simulink model "dx_hand_model"  (R2017b)
settings: Solver=ode3  StartTime=0.0  StopTime=inf  FixedStep=0.01  RelTol=1e-3  EnableMultiTasking=on
InitFcn:
  | cutFreq = 0.1; % T
  | sampleTime = 0.01;
  | filt = tf(1,[cutFreq 1]);
  | filt = c2d(filt,sampleTime);
  | 
  | cutFreq2 = 1;
  | filt2 = tf(1,[cutFreq2 1]);
  | filt2 = c2d(filt2,sampleTime);
  | 
  | cutFreq3 = 0.3;
  | filt3 = tf(1,[cutFreq3 1]);
  | filt3 = c2d(filt3,sampleTime);
  | 
  | update_param = 2;
  | 
  | ampliFactor = 1.60;
  | ampliFactorMiddle = 2.00;
  | ampliFactorDistal = 1;
  | 
  | % Set Hand Address
  | % RightHandAddress = '10.100.39.144';
  | RightHandAddress = '10.24.4.91';
  | Verosim = '10.100.39.22'
  | LeftHandAddress = '10.100.39.22'
  | 
  | max_force = 24; % Newton
model workspace (MAT data in the model file):
  SL_ROS_VariableLengthArrays_MaxSizes : struct (value not decoded)
libraries: robotlib x136, simulink_extras x27, simulink x16, etargetslib x2, dspnetwork x2
(part 2 of 19)

== system dx_hand_model/Pinky Finger/Choose_ ==
  pos : Inport
  force : Inport  Port=2
  Data Type Conversion1 : DataTypeConversion  OutDataTypeStr=single
  Get Parameter3 : robotlib/Get Parameter  SourceLibraryInfo=This block requires Robotics System Toolbox  ParameterSource=Specify your own  ParameterName=/hand_exo/pinky/modes/type  ParameterType=double  ParameterMaxArrayLength=16  ParameterInitialValue=1.0  SampleTime=update_param  ShowErrorCodeOutput=off  ModelName=dx_hand_model  BlockId=ParamGet_dx_hand_model_4579
      settings: SourceProductName=Robotics System Toolbox  SourceProductBaseCode=RO
  Rate Transition : RateTransition
  Switch : Switch  Criteria=u2 > Threshold
  out : Outport
  wires:
  Switch/1 -> out/1
  Data Type Conversion1/1 -> Switch/2
  Rate Transition/1 -> Data Type Conversion1/1
  Get Parameter3/1 -> Rate Transition/1
  force/1 -> Switch/3
  pos/1 -> Switch/1

== system dx_hand_model/Pinky Finger/Jacobian Calculation ==
  note: this jacobian has all lenght expressed in meters
  note: this jacobian has all lenght expressed in mm
  Pose : Inport
  Sensor : Inport  Port=2
  Measurements : Inport  Port=3
  Data Type Conversion1 : DataTypeConversion  OutDataTypeStr=single
  Data Type Conversion2 : DataTypeConversion  OutDataTypeStr=single
  Display1 : Display
  Display7 : Display
  Manual Switch : ManualSwitch
  Pinky Jacobian : MATLAB Function  TreatAsAtomicUnit=on  SystemSampleTime=0.01
  "Pinky Jacobian " : MATLAB Function  TreatAsAtomicUnit=on  SystemSampleTime=0.01
  Unit Delay1 : UnitDelay  InitialCondition=-1  SampleTime=0.01
  Unit Delay3 : UnitDelay  InitialCondition=[0;2.3]  SampleTime=0.01
  Jacobian : Outport
  wires:
  Pinky Jacobian/1(JTcomp) -> Manual Switch/2, Display7/1
  Data Type Conversion1/1 -> Pinky Jacobian/5(J22_old)
  Pinky Jacobian/2(q_next) -> Unit Delay3/1
  Data Type Conversion2/1 -> Pinky Jacobian/4(q_pr)
  Pinky Jacobian/3(J22_ol) -> Unit Delay1/1
  Unit Delay3/1 -> Data Type Conversion2/1
  Unit Delay1/1 -> Data Type Conversion1/1
  Measurements/1 -> "Pinky Jacobian "/3(measurements), Pinky Jacobian/3(measurements)
  Sensor/1 -> "Pinky Jacobian "/2(sensor), Pinky Jacobian/2(sensor)
  "Pinky Jacobian "/1(JTcomp) -> Display1/1, Manual Switch/1
  Pose/1 -> "Pinky Jacobian "/1(pose), Pinky Jacobian/1(pose)
  Manual Switch/1 -> Jacobian/1

== system dx_hand_model/Pinky Finger/Pose Generator ==
  Angular Potentiometer : Subsystem
  Constant : Constant
  Constant3 : Constant  Value=0
  Display : Display
  Display1 : Display
  Display3 : Display
  Linear Potentiometer : Subsystem
  Manual Switch : ManualSwitch  CurrentSetting=0
  Mux1 : Mux  Inputs=2
  Parametri Ring : Subsystem
  Pinky Direct Kinematics : MATLAB Function  TreatAsAtomicUnit=on
  Pinky Parameters : Subsystem
  Rate Transition : RateTransition
  Record : Subsystem
  Saturation2 : Saturate  UpperLimit=1000  LowerLimit=0
  Saturation3 : Saturate  UpperLimit=1000  LowerLimit=0
  Pose : Outport
  Sensors : Outport  Port=2
  Measurements : Outport  Port=3
  tag scope: PinkyPot1=global
  wires:
  Pinky Direct Kinematics/1(y) -> Pose/1, Record/3(output)
  Manual Switch/1 -> Record/Enable
  Angular Potentiometer/1(Deg) -> Display3/1
  [PinkyRotPot] -> Angular Potentiometer/1(ADC)
  [PinkyFlexLinPot] -> Linear Potentiometer/1(ADC)
  Saturation2/1 -> [PinkyPot1], Mux1/1
  Constant/1 -> Manual Switch/1
  Constant3/1 -> Manual Switch/2
  Angular Potentiometer/2(Rad) -> Display1/1, Saturation3/1
  Linear Potentiometer/1(mm) -> Display/1, Saturation2/1
  Mux1/1 -> Sensors/1, Record/1(input), Pinky Direct Kinematics/1(u)
  Saturation3/1 -> Mux1/2
  Pinky Parameters/1(to Direct Kin) -> Pinky Direct Kinematics/2(measurements), Measurements/1, Record/2(param)
  Parametri Ring/1(Par_5) -> Rate Transition/1
  Rate Transition/1 -> Pinky Parameters/1(Par5)

== system dx_hand_model/Pinky Finger/Position-Force Architecture ==
  Jacobian : Inport
  Classic_Static_Problem : MATLAB Function  TreatAsAtomicUnit=on
  Display6 : Display
  Optimized_Static_Problem : MATLAB Function  TreatAsAtomicUnit=on
  Position Force Basic Architecture : Subsystem
  Subsystem : Subsystem
  Feedforward Force : Outport
  wires:
  Position Force Basic Architecture/1(force_vec) -> Classic_Static_Problem/2(force_vector), Optimized_Static_Problem/2(force_vector)
  Jacobian/1 -> Classic_Static_Problem/1(Jcomponents), Optimized_Static_Problem/1(Jcomponents)
  Subsystem/1(J_out) -> Feedforward Force/1, Display6/1
  Optimized_Static_Problem/1(y) -> Subsystem/1(optim)
  Classic_Static_Problem/1(y) -> Subsystem/2(classic)

== system dx_hand_model/Pinky Finger/Position-Position ==
  Jacobian : Inport
  Classic_Static_Problem : MATLAB Function  TreatAsAtomicUnit=on
  Discrete Derivative{,1..3} (4 alike) : simulink/Discrete/Discrete Derivative  gainval=1.0  ICPrevScaledInput=0.0  OutMin=[]  OutMax=[]  OutDataType=fixdt(1, 16)  OutScaling=2^-10  DoSatur=off
  Gain : Gain  Gain=1.3588
  Mux : Mux  Inputs=2
  Mux1 : Mux  Inputs=2
  Optimized_Static_Problem : MATLAB Function  TreatAsAtomicUnit=on
  Pre-Proc : Subsystem
  Saturation3 : Saturate  UpperLimit=0.80  LowerLimit=0
  Saturation4 : Saturate  UpperLimit=1.33  LowerLimit=0
  Sum{,1,3..4} (4 alike) : Sum  Inputs=|+-
  Sum2 : Sum  Inputs=|++
  active : Subsystem
  active1 : Subsystem
  setGain : Subsystem
  "setGain " : Subsystem
  setGain 1 : Subsystem
  setGain 2 : Subsystem
  rate : Outport
  wires:
  [act_Pinky] -> Gain/1, Discrete Derivative2/1, Sum/1
  Sum/1 -> setGain/1(in)
  "setGain "/1(out) -> Mux/2
  setGain/1(out) -> Mux/1
  [SchunkPinkyFingerDistal] -> Saturation4/1
  Mux/1 -> Sum2/1
  Mux1/1 -> Sum2/2
  Sum2/1 -> Optimized_Static_Problem/2(force_vector), Classic_Static_Problem/2(operational_space)
  [SchunkPinkyFingerProximal] -> Saturation3/1
  Saturation3/1 -> Sum/2, Discrete Derivative/1
  Saturation4/1 -> Sum1/2, Discrete Derivative1/1
  Gain/1 -> Discrete Derivative3/1, Sum1/1
  Jacobian/1 -> Optimized_Static_Problem/1(Jcomponents), Classic_Static_Problem/1(Jcomponents)
  Sum1/1 -> "setGain "/1(in)
  Sum3/1 -> setGain 1/1(in)
  Sum4/1 -> setGain 2/1(in)
  setGain 1/1(out) -> Mux1/1
  setGain 2/1(out) -> Mux1/2
  Optimized_Static_Problem/1(y) -> Pre-Proc/1(yes)
  Classic_Static_Problem/1(rate) -> Pre-Proc/2(no)
  Pre-Proc/1(out) -> rate/1
  Discrete Derivative/1 -> Sum3/2
  Discrete Derivative1/1 -> Sum4/2
  Discrete Derivative2/1 -> active/1(in)
  active/1(out) -> Sum3/1
  Discrete Derivative3/1 -> active1/1(in)
  active1/1(out) -> Sum4/1

== system dx_hand_model/Pinky Finger/Pre-Proc ==
  in : Inport
  Data Type Conversion1 : DataTypeConversion  OutDataTypeStr=single
  Data Type Conversion2 : DataTypeConversion  OutDataTypeStr=single
  Filt 4 : DiscreteTransferFcn  Numerator=filt2.Numerator{1,1}  Denominator=filt2.Denominator{1,1}  SampleTime=0.01
  Get Parameter3 : robotlib/Get Parameter  SourceLibraryInfo=This block requires Robotics System Toolbox  ParameterSource=Specify your own  ParameterName=/hand_exo/pinky/j_f  ParameterType=double  ParameterMaxArrayLength=16  ParameterInitialValue=1.0  SampleTime=update_param  ShowErrorCodeOutput=on  ModelName=dx_hand_model  BlockId=ParamGet_dx_hand_model_4804
      settings: SourceProductName=Robotics System Toolbox  SourceProductBaseCode=RO
  "IsNan " : MATLAB Function  TreatAsAtomicUnit=on
  Memory : Memory  InitialCondition=[0,0,0,0]
  Rate Transition : RateTransition
  Switch : Switch  Criteria=u2 > Threshold
  out : Outport
  wires:
  Get Parameter3/1 -> Rate Transition/1
  Rate Transition/1 -> Data Type Conversion1/1
  Data Type Conversion1/1 -> Switch/2
  Filt 4/1 -> Switch/1
  Switch/1 -> out/1
  Memory/1 -> Data Type Conversion2/1
  in/1 -> "IsNan "/1(Jin)
  Data Type Conversion2/1 -> "IsNan "/2(J_k1)
  "IsNan "/1(J) -> Switch/3, Filt 4/1, Memory/1

== system dx_hand_model/Pinky Finger/setGain ==
  in : Inport
  Data Type Conversion1 : DataTypeConversion  OutDataTypeStr=single
  Get Parameter3 : robotlib/Get Parameter  SourceLibraryInfo=This block requires Robotics System Toolbox  ParameterSource=Specify your own  ParameterName=/hand_exo/pinky/schunk_gains/prox  ParameterType=double  ParameterMaxArrayLength=16  ParameterInitialValue=1.0  SampleTime=update_param  ShowErrorCodeOutput=off  ModelName=dx_hand_model  BlockId=ParamGet_dx_hand_model_4815
      settings: SourceProductName=Robotics System Toolbox  SourceProductBaseCode=RO
  Product : Product
  Rate Transition : RateTransition
  out : Outport
  wires:
  Product/1 -> out/1
  Data Type Conversion1/1 -> Product/1
  in/1 -> Product/2
  Rate Transition/1 -> Data Type Conversion1/1
  Get Parameter3/1 -> Rate Transition/1

== system dx_hand_model/Pinky Finger/setGain1 ==
  in : Inport
  Data Type Conversion1 : DataTypeConversion  OutDataTypeStr=single
  Get Parameter3 : robotlib/Get Parameter  SourceLibraryInfo=This block requires Robotics System Toolbox  ParameterSource=Specify your own  ParameterName=/hand_exo/pinky/schunk_gains/dist  ParameterType=double  ParameterMaxArrayLength=16  ParameterInitialValue=1.0  SampleTime=update_param  ShowErrorCodeOutput=off  ModelName=dx_hand_model  BlockId=ParamGet_dx_hand_model_4822
      settings: SourceProductName=Robotics System Toolbox  SourceProductBaseCode=RO
  Product : Product
  Rate Transition : RateTransition
  out : Outport
  wires:
  Product/1 -> out/1
  Data Type Conversion1/1 -> Product/1
  in/1 -> Product/2
  Rate Transition/1 -> Data Type Conversion1/1
  Get Parameter3/1 -> Rate Transition/1

== system dx_hand_model/Pinky Finger/setGain2 ==
  in : Inport
  Data Type Conversion1 : DataTypeConversion  OutDataTypeStr=single
  Get Parameter3 : robotlib/Get Parameter  SourceLibraryInfo=This block requires Robotics System Toolbox  ParameterSource=Specify your own  ParameterName=/hand_exo/pinky/modes/saturator  ParameterType=double  ParameterMaxArrayLength=16  ParameterInitialValue=-1.0  SampleTime=update_param  ShowErrorCodeOutput=off  ModelName=dx_hand_model  BlockId=ParamGet_dx_hand_model_4829
      settings: SourceProductName=Robotics System Toolbox  SourceProductBaseCode=RO
  Rate Transition : RateTransition
  Saturation1 : Saturate  UpperLimit=max_force  LowerLimit=-max_force
  Saturation2 : Saturate  UpperLimit=0  LowerLimit=-max_force
  Switch : Switch  Criteria=u2 > Threshold
  out : Outport
  wires:
  Switch/1 -> out/1
  Data Type Conversion1/1 -> Switch/2
  Rate Transition/1 -> Data Type Conversion1/1
  Get Parameter3/1 -> Rate Transition/1
  in/1 -> Saturation1/1, Saturation2/1
  Saturation1/1 -> Switch/1
  Saturation2/1 -> Switch/3

== system dx_hand_model/Ring Finger /Active ==
  in : Inport
  Constant : Constant  Value=0  OutDataTypeStr=single
  Data Type Conversion1 : DataTypeConversion  OutDataTypeStr=single
  Get Parameter3 : robotlib/Get Parameter  SourceLibraryInfo=This block requires Robotics System Toolbox  ParameterSource=Specify your own  ParameterName=/hand_exo/ring/modes/ff_active  ParameterType=double  ParameterMaxArrayLength=16  ParameterInitialValue=1.0  SampleTime=update_param  ShowErrorCodeOutput=off  ModelName=dx_hand_model  BlockId=ParamGet_dx_hand_model_4879
      settings: SourceProductName=Robotics System Toolbox  SourceProductBaseCode=RO
  Rate Transition : RateTransition
  Switch : Switch  Criteria=u2 > Threshold
  out : Outport
  wires:
  Switch/1 -> out/1
  Data Type Conversion1/1 -> Switch/2
  Rate Transition/1 -> Data Type Conversion1/1
  Get Parameter3/1 -> Rate Transition/1
  in/1 -> Switch/1
  Constant/1 -> Switch/3

== system dx_hand_model/Ring Finger /Choose ==
  theoretical : Inport
  empiric : Inport  Port=2
  Data Type Conversion1 : DataTypeConversion  OutDataTypeStr=single
  Get Parameter3 : robotlib/Get Parameter  SourceLibraryInfo=This block requires Robotics System Toolbox  ParameterSource=Specify your own  ParameterName=/hand_exo/ring/modes/theor  ParameterType=double  ParameterMaxArrayLength=16  ParameterInitialValue=-1.0  SampleTime=update_param  ShowErrorCodeOutput=off  ModelName=dx_hand_model  BlockId=ParamGet_dx_hand_model_4903
      settings: SourceProductName=Robotics System Toolbox  SourceProductBaseCode=RO
  Rate Transition : RateTransition
  Switch : Switch  Criteria=u2 > Threshold
  out : Outport
  wires:
  Switch/1 -> out/1
  Data Type Conversion1/1 -> Switch/2
  Rate Transition/1 -> Data Type Conversion1/1
  Get Parameter3/1 -> Rate Transition/1
  empiric/1 -> Switch/3
  theoretical/1 -> Switch/1

== system dx_hand_model/Ring Finger /Choose_ ==
  pos : Inport
  force : Inport  Port=2
  Data Type Conversion1 : DataTypeConversion  OutDataTypeStr=single
  Get Parameter3 : robotlib/Get Parameter  SourceLibraryInfo=This block requires Robotics System Toolbox  ParameterSource=Specify your own  ParameterName=/hand_exo/ring/modes/type  ParameterType=double  ParameterMaxArrayLength=16  ParameterInitialValue=1.0  SampleTime=update_param  ShowErrorCodeOutput=off  ModelName=dx_hand_model  BlockId=ParamGet_dx_hand_model_4283
      settings: SourceProductName=Robotics System Toolbox  SourceProductBaseCode=RO
  Rate Transition : RateTransition
  Switch : Switch  Criteria=u2 > Threshold
  out : Outport
  wires:
  Switch/1 -> out/1
  Data Type Conversion1/1 -> Switch/2
  Rate Transition/1 -> Data Type Conversion1/1
  Get Parameter3/1 -> Rate Transition/1
  force/1 -> Switch/3
  pos/1 -> Switch/1

== system dx_hand_model/Ring Finger /Jacobian Calculation ==
  note: this jacobian has all lenght expressed in meters
  note: this jacobian has all lenght expressed in mm
  Pose : Inport
  Sensor : Inport  Port=2
  Measurements : Inport  Port=3
  Data Type Conversion1 : DataTypeConversion  OutDataTypeStr=single
  Data Type Conversion2 : DataTypeConversion  OutDataTypeStr=single
  Display1 : Display
  Display7 : Display
  Manual Switch : ManualSwitch
  Ring Jacobian : MATLAB Function  TreatAsAtomicUnit=on  SystemSampleTime=0.01
  "Ring Jacobian " : MATLAB Function  TreatAsAtomicUnit=on  SystemSampleTime=0.01
  Unit Delay1 : UnitDelay  InitialCondition=-1  SampleTime=0.01
  Unit Delay3 : UnitDelay  InitialCondition=[0;2.3]  SampleTime=0.01
  Jacobian : Outport
  wires:
  Ring Jacobian/1(JTcomp) -> Manual Switch/2, Display7/1
  Data Type Conversion1/1 -> Ring Jacobian/5(J22_old)
  Ring Jacobian/2(q_next) -> Unit Delay3/1
  Data Type Conversion2/1 -> Ring Jacobian/4(q_pr)
  Ring Jacobian/3(J22_ol) -> Unit Delay1/1
  Unit Delay3/1 -> Data Type Conversion2/1
  Unit Delay1/1 -> Data Type Conversion1/1
  Measurements/1 -> "Ring Jacobian "/3(measurements), Ring Jacobian/3(measurements)
  Sensor/1 -> "Ring Jacobian "/2(sensor), Ring Jacobian/2(sensor)
  "Ring Jacobian "/1(JTcomp) -> Display1/1, Manual Switch/1
  Pose/1 -> "Ring Jacobian "/1(pose), Ring Jacobian/1(pose)
  Manual Switch/1 -> Jacobian/1

== system dx_hand_model/Ring Finger /Pose Generator ==
  Angular Potentiometer : Subsystem
  Constant : Constant
  Constant3 : Constant  Value=0
  Display : Display
  Display1 : Display
  Display3 : Display
  Linear Potentiometer : Subsystem
  Manual Switch : ManualSwitch  CurrentSetting=0
  Mux1 : Mux  Inputs=2
  Parametri Ring : Subsystem
  Rate Transition : RateTransition
  Record : Subsystem
  Ring Direct Kinematics : MATLAB Function  TreatAsAtomicUnit=on
  Ring Parameters : Subsystem
  Saturation2 : Saturate  UpperLimit=1000  LowerLimit=0
  Saturation3 : Saturate  UpperLimit=1000  LowerLimit=0
  Pose : Outport
  Sensors : Outport  Port=2
  Measurements : Outport  Port=3
  tag scope: RingPot1=global
  wires:
  Ring Direct Kinematics/1(y) -> Pose/1, Record/3(output)
  Manual Switch/1 -> Record/Enable
  Angular Potentiometer/1(Deg) -> Display3/1
  [RingRotPot] -> Angular Potentiometer/1(ADC)
  [RingFlexLinPot] -> Linear Potentiometer/1(ADC)
  Saturation2/1 -> [RingPot1], Mux1/1
  Constant/1 -> Manual Switch/1
  Constant3/1 -> Manual Switch/2
  Angular Potentiometer/2(Rad) -> Display1/1, Saturation3/1
  Linear Potentiometer/1(mm) -> Display/1, Saturation2/1
  Mux1/1 -> Sensors/1, Record/1(input), Ring Direct Kinematics/1(u)
  Saturation3/1 -> Mux1/2
  Ring Parameters/1(to Direct Kin) -> Ring Direct Kinematics/2(measurements), Measurements/1, Record/2(param)
  Parametri Ring/1(Par_5) -> Rate Transition/1
  Rate Transition/1 -> Ring Parameters/1(Par5)

== system dx_hand_model/Ring Finger /Position-Force Architecture ==
  Jacobian : Inport
  Classic_Static_Problem : MATLAB Function  TreatAsAtomicUnit=on
  Display6 : Display
  Optimized_Static_Problem : MATLAB Function  TreatAsAtomicUnit=on
  Position Force Basic Architecture : Subsystem
  Subsystem : Subsystem
  Feedforward Force : Outport
  wires:
  Position Force Basic Architecture/1(force_vec) -> Classic_Static_Problem/2(force_vector), Optimized_Static_Problem/2(force_vector)
  Jacobian/1 -> Classic_Static_Problem/1(Jcomponents), Optimized_Static_Problem/1(Jcomponents)
  Subsystem/1(J_out) -> Feedforward Force/1, Display6/1
  Optimized_Static_Problem/1(y) -> Subsystem/1(optim)
  Classic_Static_Problem/1(y) -> Subsystem/2(classic)

== system dx_hand_model/Ring Finger /Position-Position ==
  Jacobian : Inport
  Classic_Static_Problem : MATLAB Function  TreatAsAtomicUnit=on
  Discrete Derivative{,1..3} (4 alike) : simulink/Discrete/Discrete Derivative  gainval=1.0  ICPrevScaledInput=0.0  OutMin=[]  OutMax=[]  OutDataType=fixdt(1, 16)  OutScaling=2^-10  DoSatur=off
  Gain : Gain  Gain=1.3588
  Mux : Mux  Inputs=2
  Mux1 : Mux  Inputs=2
  Optimized_Static_Problem : MATLAB Function  TreatAsAtomicUnit=on
  Pre-Proc : Subsystem
  Saturation3 : Saturate  UpperLimit=0.80  LowerLimit=0
  Saturation4 : Saturate  UpperLimit=1.33  LowerLimit=0
  Sum{,1,3..4} (4 alike) : Sum  Inputs=|+-
  Sum2 : Sum  Inputs=|++
  active : Subsystem
  active1 : Subsystem
  setGain : Subsystem
  "setGain " : Subsystem
  setGain 1 : Subsystem
  setGain 2 : Subsystem
  rate : Outport
  wires:
  [act_Ring] -> Gain/1, Discrete Derivative2/1, Sum/1
  Sum/1 -> setGain/1(in)
  "setGain "/1(out) -> Mux/2
  setGain/1(out) -> Mux/1
  [SchunkRingFingerDistal] -> Saturation4/1
  Mux/1 -> Sum2/1
  Mux1/1 -> Sum2/2
  Sum2/1 -> Optimized_Static_Problem/2(force_vector), Classic_Static_Problem/2(operational_space)
  [SchunkRingFingerProximal] -> Saturation3/1
  Saturation3/1 -> Sum/2, Discrete Derivative/1
  Saturation4/1 -> Sum1/2, Discrete Derivative1/1
  Gain/1 -> Discrete Derivative3/1, Sum1/1
  Jacobian/1 -> Optimized_Static_Problem/1(Jcomponents), Classic_Static_Problem/1(Jcomponents)
  Sum1/1 -> "setGain "/1(in)
  Sum3/1 -> setGain 1/1(in)
  Sum4/1 -> setGain 2/1(in)
  setGain 1/1(out) -> Mux1/1
  setGain 2/1(out) -> Mux1/2
  Optimized_Static_Problem/1(y) -> Pre-Proc/1(yes)
  Classic_Static_Problem/1(rate) -> Pre-Proc/2(no)
  Pre-Proc/1(out) -> rate/1
  Discrete Derivative/1 -> Sum3/2
  Discrete Derivative1/1 -> Sum4/2
  Discrete Derivative2/1 -> active/1(in)
  active/1(out) -> Sum3/1
  Discrete Derivative3/1 -> active1/1(in)
  active1/1(out) -> Sum4/1

== system dx_hand_model/Ring Finger /Pre-Proc ==
  in : Inport
  Data Type Conversion1 : DataTypeConversion  OutDataTypeStr=single
  Data Type Conversion2 : DataTypeConversion  OutDataTypeStr=single
  Filt 4 : DiscreteTransferFcn  Numerator=filt2.Numerator{1,1}  Denominator=filt2.Denominator{1,1}  SampleTime=0.01
  Get Parameter3 : robotlib/Get Parameter  SourceLibraryInfo=This block requires Robotics System Toolbox  ParameterSource=Specify your own  ParameterName=/hand_exo/ring/j_f  ParameterType=double  ParameterMaxArrayLength=16  ParameterInitialValue=1.0  SampleTime=update_param  ShowErrorCodeOutput=on  ModelName=dx_hand_model  BlockId=ParamGet_dx_hand_model_4518
      settings: SourceProductName=Robotics System Toolbox  SourceProductBaseCode=RO
  "IsNan " : MATLAB Function  TreatAsAtomicUnit=on
  Memory : Memory  InitialCondition=[0,0,0,0]
  Rate Transition : RateTransition
  Switch : Switch  Criteria=u2 > Threshold
  out : Outport
  wires:
  Get Parameter3/1 -> Rate Transition/1
  Rate Transition/1 -> Data Type Conversion1/1
  Data Type Conversion1/1 -> Switch/2
  Filt 4/1 -> Switch/1
  Switch/1 -> out/1
  Memory/1 -> Data Type Conversion2/1
  in/1 -> "IsNan "/1(Jin)
  Data Type Conversion2/1 -> "IsNan "/2(J_k1)
  "IsNan "/1(J) -> Switch/3, Filt 4/1, Memory/1

== system dx_hand_model/Ring Finger /setGain ==
  in : Inport
  Data Type Conversion1 : DataTypeConversion  OutDataTypeStr=single
  Get Parameter3 : robotlib/Get Parameter  SourceLibraryInfo=This block requires Robotics System Toolbox  ParameterSource=Specify your own  ParameterName=/hand_exo/ring/schunk_gains/prox  ParameterType=double  ParameterMaxArrayLength=16  ParameterInitialValue=1.0  SampleTime=update_param  ShowErrorCodeOutput=off  ModelName=dx_hand_model  BlockId=ParamGet_dx_hand_model_4529
      settings: SourceProductName=Robotics System Toolbox  SourceProductBaseCode=RO
  Product : Product
  Rate Transition : RateTransition
  out : Outport
  wires:
  Product/1 -> out/1
  Data Type Conversion1/1 -> Product/1
  in/1 -> Product/2
  Rate Transition/1 -> Data Type Conversion1/1
  Get Parameter3/1 -> Rate Transition/1

== system dx_hand_model/Ring Finger /setGain1 ==
  in : Inport
  Data Type Conversion1 : DataTypeConversion  OutDataTypeStr=single
  Get Parameter3 : robotlib/Get Parameter  SourceLibraryInfo=This block requires Robotics System Toolbox  ParameterSource=Specify your own  ParameterName=/hand_exo/ring/schunk_gains/dist  ParameterType=double  ParameterMaxArrayLength=16  ParameterInitialValue=1.0  SampleTime=update_param  ShowErrorCodeOutput=off  ModelName=dx_hand_model  BlockId=ParamGet_dx_hand_model_4536
      settings: SourceProductName=Robotics System Toolbox  SourceProductBaseCode=RO
  Product : Product
  Rate Transition : RateTransition
  out : Outport
  wires:
  Product/1 -> out/1
  Data Type Conversion1/1 -> Product/1
  in/1 -> Product/2
  Rate Transition/1 -> Data Type Conversion1/1
  Get Parameter3/1 -> Rate Transition/1

== system dx_hand_model/Ring Finger /setGain2 ==
  in : Inport
  Data Type Conversion1 : DataTypeConversion  OutDataTypeStr=single
  Get Parameter3 : robotlib/Get Parameter  SourceLibraryInfo=This block requires Robotics System Toolbox  ParameterSource=Specify your own  ParameterName=/hand_exo/ring/modes/saturator  ParameterType=double  ParameterMaxArrayLength=16  ParameterInitialValue=-1.0  SampleTime=update_param  ShowErrorCodeOutput=off  ModelName=dx_hand_model  BlockId=ParamGet_dx_hand_model_4543
      settings: SourceProductName=Robotics System Toolbox  SourceProductBaseCode=RO
  Rate Transition : RateTransition
  Saturation1 : Saturate  UpperLimit=max_force  LowerLimit=-max_force
  Saturation2 : Saturate  UpperLimit=0  LowerLimit=-max_force
  Switch : Switch  Criteria=u2 > Threshold
  out : Outport
  wires:
  Switch/1 -> out/1
  Data Type Conversion1/1 -> Switch/2
  Rate Transition/1 -> Data Type Conversion1/1
  Get Parameter3/1 -> Rate Transition/1
  in/1 -> Saturation1/1, Saturation2/1
  Saturation1/1 -> Switch/1
  Saturation2/1 -> Switch/3

== system dx_hand_model/Send to Schunk/Enable ==
  "Automatic " : ManualSwitch  CurrentSetting=0
  Blank Message1 : robotlib/Blank Message  SourceLibraryInfo=This block requires Robotics System Toolbox  messageType=std_msgs/Bool  SampleTime=inf
      settings: SourceProductBaseCode=RO
  Bus Assignment2 : BusAssignment  AssignedSignals=Data
  Bus Selector : BusSelector  OutputSignals=Data
  Constant : Constant  Value=0  OutDataTypeStr=boolean
  Constant1 : Constant  OutDataTypeStr=boolean
  Logical Operator : Logic  Operator=NOT  AllPortsSameDT=off  OutDataTypeStr=boolean
  Logical Operator1 : Logic  AllPortsSameDT=off  OutDataTypeStr=boolean
  Manual Switch : ManualSwitch  CurrentSetting=0
  Publish2 : robotlib/Publish  SourceLibraryInfo=This block requires Robotics System Toolbox  topicSource=Specify your own  topic=/trigger_exo_hand  messageType=std_msgs/Bool  messageQueueLength=1
      settings: SourceProductBaseCode=RO
  Subscribe : robotlib/Subscribe  SourceLibraryInfo=This block requires Robotics System Toolbox  topicSource=Specify your own  topic=/manual_commands/start  messageType=std_msgs/Bool  sampleTime=0.01  messageQueueLength=1
      settings: SourceProductBaseCode=RO
  Terminator : Terminator
  wires:
  Bus Assignment2/1 -> Publish2/1
  [CalibrationSignal] -> Logical Operator/1
  Manual Switch/1 -> "Automatic "/2
  Blank Message1/1 -> Bus Assignment2/1
  Constant/1 -> Manual Switch/1
  "Automatic "/1 -> Bus Assignment2/2
  Constant1/1 -> Manual Switch/2
  Logical Operator/1 -> Logical Operator1/2
  Logical Operator1/1 -> "Automatic "/1
  Bus Selector/1 -> Logical Operator1/1  "<Data>"
  Subscribe/1 -> Terminator/1
  Subscribe/2 -> Bus Selector/1

== system dx_hand_model/Send to Schunk/Send data to Ros ==
  status : Inport
  data : Inport  Port=2
  Blank Message2 : robotlib/Blank Message  SourceLibraryInfo=This block requires Robotics System Toolbox  messageType=sensor_msgs/JointState  SampleTime=inf
      settings: SourceProductBaseCode=RO
  Data Type Conversion : DataTypeConversion  OutDataTypeStr=uint32
  MATLAB Function - Assign : MATLAB Function  TreatAsAtomicUnit=on
  Publish1 : robotlib/Publish  SourceLibraryInfo=This block requires Robotics System Toolbox  topicSource=Select from ROS network  topic=/svh_controller/channel_targets  messageType=sensor_msgs/JointState  messageQueueLength=1
      settings: SourceProductBaseCode=RO
  Publish12 : robotlib/Publish  Commented=on  SourceLibraryInfo=This block requires Robotics System Toolbox  topicSource=Specify your own  topic=/scan  messageType=sensor_msgs/JointState  messageQueueLength=1
      settings: SourceProductBaseCode=RO
  zzz3 : Subsystem  TreatAsAtomicUnit=on
      settings: OpenFcn=% no-op
      mask Display: disp('')
  wires:
  data/1 -> MATLAB Function - Assign/2(u)
  Blank Message2/1 -> MATLAB Function - Assign/1(blankMessage)
  Data Type Conversion/1 -> MATLAB Function - Assign/3(timeStamp)
  status/1 -> Data Type Conversion/1
  MATLAB Function - Assign/1(msg) -> Publish1/1, Publish12/1
  [SecTS] -> MATLAB Function - Assign/4(sec)
  [NSecTS] -> MATLAB Function - Assign/5(Nsec)

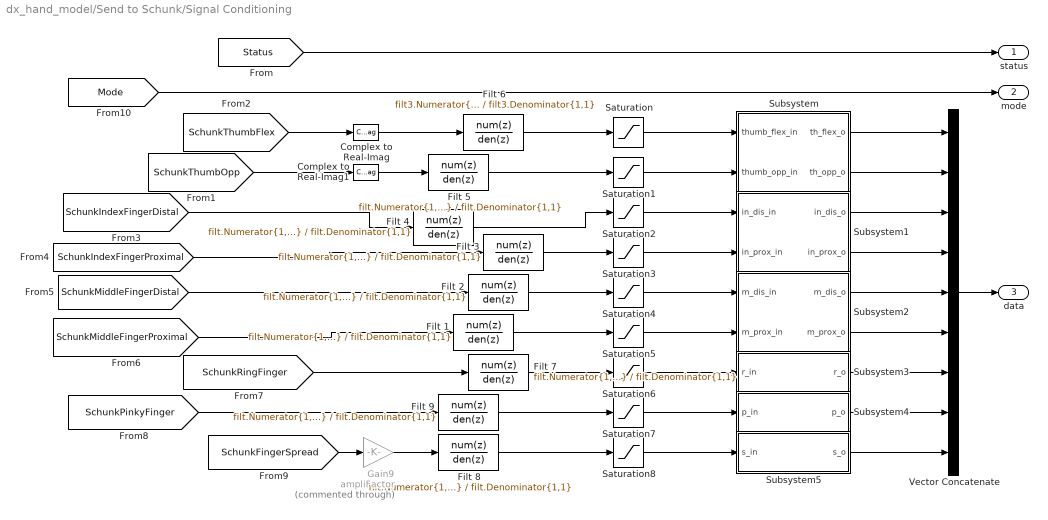
== system dx_hand_model/Send to Schunk/Signal Conditioning ==
  Complex to Real-Imag : ComplexToRealImag  Output=Real
  Complex to Real-Imag1 : ComplexToRealImag  Output=Real
  Filt {1..5,7..9} (8 alike) : DiscreteTransferFcn  Numerator=filt.Numerator{1,1}  Denominator=filt.Denominator{1,1}  SampleTime=0.01
  Filt 6 : DiscreteTransferFcn  Numerator=filt3.Numerator{1,1}  Denominator=filt3.Denominator{1,1}  SampleTime=0.01
  Gain9 : Gain  Commented=through  Gain=ampliFactor
  Saturation : Saturate  UpperLimit=0.97  LowerLimit=0
  Saturation1 : Saturate  UpperLimit=0.99  LowerLimit=0
  Saturation2 : Saturate  UpperLimit=1.33  LowerLimit=0
  Saturation3 : Saturate  UpperLimit=0.80  LowerLimit=0
  Saturation4 : Saturate  UpperLimit=1.33  LowerLimit=0
  Saturation5 : Saturate  UpperLimit=0.80  LowerLimit=0
  Saturation6 : Saturate  UpperLimit=0.98  LowerLimit=0
  Saturation7 : Saturate  UpperLimit=0.98  LowerLimit=0
  Saturation8 : Saturate  UpperLimit=0.30  LowerLimit=0.05
  Subsystem : Subsystem
  Subsystem1 : Subsystem
  Subsystem2 : Subsystem
  Subsystem3 : Subsystem
  Subsystem4 : Subsystem
  Subsystem5 : Subsystem
  Vector Concatenate : Concatenate  NumInputs=9
  status : Outport
  mode : Outport  Port=2
  data : Outport  Port=3
  wires:
  [SchunkMiddleFingerProximal] -> Filt 1/1
  [SchunkIndexFingerProximal] -> Filt 3/1
  [SchunkIndexFingerDistal] -> Filt 4/1
  [SchunkMiddleFingerDistal] -> Filt 2/1
  Filt 8/1 -> Saturation8/1
  [SchunkThumbOpp] -> Complex to Real-Imag1/1
  [SchunkFingerSpread] -> Gain9/1
  [SchunkPinkyFinger] -> Filt 9/1
  [SchunkRingFinger] -> Filt 7/1
  Gain9/1 -> Filt 8/1
  [Mode] -> mode/1
  [Status] -> status/1
  Saturation8/1 -> Subsystem5/1(s_in)
  Saturation6/1 -> Subsystem3/1(r_in)
  Saturation7/1 -> Subsystem4/1(p_in)
  [SchunkThumbFlex] -> Complex to Real-Imag/1
  Subsystem/1(th_flex_o) -> Vector Concatenate/1
  Subsystem/2(th_opp_o) -> Vector Concatenate/2
  Subsystem1/1(in_dis_o) -> Vector Concatenate/3
  Subsystem1/2(in_prox_o) -> Vector Concatenate/4
  Subsystem2/1(m_dis_o) -> Vector Concatenate/5
  Subsystem2/2(m_prox_o) -> Vector Concatenate/6
  Subsystem3/1(r_o) -> Vector Concatenate/7
  Subsystem4/1(p_o) -> Vector Concatenate/8
  Subsystem5/1(s_o) -> Vector Concatenate/9
  Vector Concatenate/1 -> data/1
  Saturation4/1 -> Subsystem2/1(m_dis_in)
  Saturation5/1 -> Subsystem2/2(m_prox_in)
  Saturation1/1 -> Subsystem/2(thumb_opp_in)
  Saturation/1 -> Subsystem/1(thumb_flex_in)
  Saturation2/1 -> Subsystem1/1(in_dis_in)
  Saturation3/1 -> Subsystem1/2(in_prox_in)
  Filt 1/1 -> Saturation5/1
  Filt 2/1 -> Saturation4/1
  Filt 3/1 -> Saturation3/1
  Filt 4/1 -> Saturation2/1
  Filt 5/1 -> Saturation1/1
  Filt 6/1 -> Saturation/1
  Complex to Real-Imag/1 -> Filt 6/1
  Complex to Real-Imag1/1 -> Filt 5/1
  Filt 7/1 -> Saturation6/1
  Filt 9/1 -> Saturation7/1

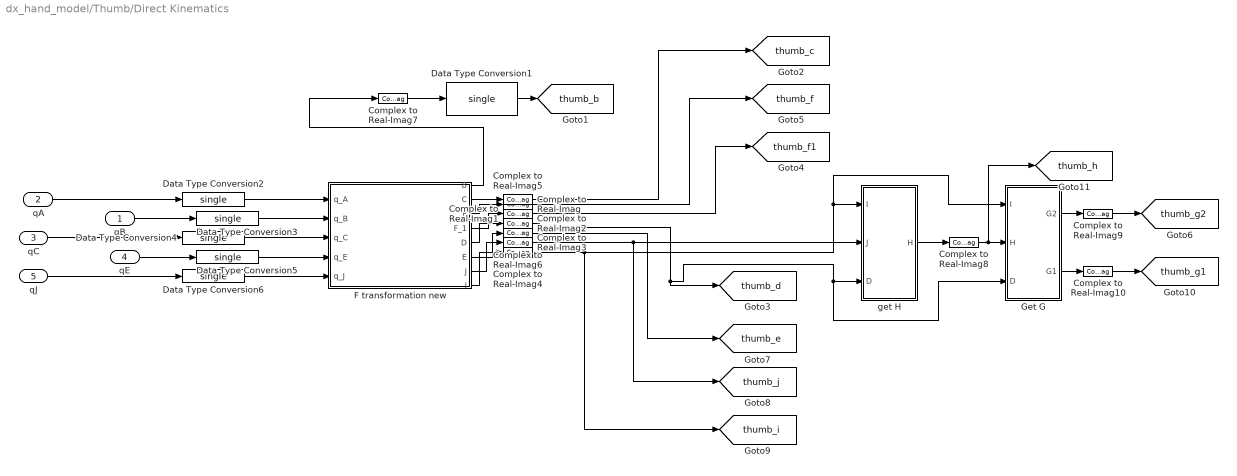
== system dx_hand_model/Thumb/Direct Kinematics ==
  qB : Inport
  qA : Inport  Port=2
  qC : Inport  Port=3
  qE : Inport  Port=4
  qJ : Inport  Port=5
  Complex to Real-Imag{,1..10} (11 alike) : ComplexToRealImag  Output=Real
  Data Type Conversion{1..6} (6 alike) : DataTypeConversion  OutDataTypeStr=single
  F transformation new : MATLAB Function  TreatAsAtomicUnit=on
  Get G : Subsystem
  get H : Subsystem
  tag scope: thumb_b=global, thumb_c=global, thumb_d=global, thumb_e=global, thumb_f1=global, thumb_f=global, thumb_g1=global, thumb_g2=global, thumb_h=global, thumb_i=global, thumb_j=global
  wires:
  Complex to Real-Imag5/1 -> [thumb_c]
  qA/1 -> Data Type Conversion2/1
  Complex to Real-Imag6/1 -> [thumb_e]
  F transformation new/6(E) -> Complex to Real-Imag6/1
  F transformation new/1(B) -> Complex to Real-Imag7/1
  qE/1 -> Data Type Conversion5/1
  qB/1 -> Data Type Conversion3/1
  qC/1 -> Data Type Conversion4/1
  F transformation new/3(F) -> Complex to Real-Imag/1
  F transformation new/4(F_1) -> Complex to Real-Imag1/1
  F transformation new/7(J) -> Complex to Real-Imag3/1
  F transformation new/8(I) -> Complex to Real-Imag4/1
  F transformation new/5(D) -> Complex to Real-Imag2/1
  Complex to Real-Imag/1 -> [thumb_f]
  Complex to Real-Imag1/1 -> [thumb_f1]
  F transformation new/2(C) -> Complex to Real-Imag5/1
  Complex to Real-Imag7/1 -> Data Type Conversion1/1
  Data Type Conversion1/1 -> [thumb_b]
  Data Type Conversion2/1 -> F transformation new/1(q_A)
  Data Type Conversion3/1 -> F transformation new/2(q_B)
  Data Type Conversion4/1 -> F transformation new/3(q_C)
  Data Type Conversion5/1 -> F transformation new/4(q_E)
  Data Type Conversion6/1 -> F transformation new/5(q_J)
  qJ/1 -> Data Type Conversion6/1
  Complex to Real-Imag4/1 -> [thumb_i], Get G/1(I), get H/1(I)
  Complex to Real-Imag2/1 -> [thumb_d], Get G/3(D), get H/3(D)
  Get G/1(G2) -> Complex to Real-Imag9/1
  Get G/2(G1) -> Complex to Real-Imag10/1
  get H/1(H) -> Complex to Real-Imag8/1
  Complex to Real-Imag3/1 -> get H/2(J), [thumb_j]
  Complex to Real-Imag8/1 -> [thumb_h], Get G/2(H)
  Complex to Real-Imag9/1 -> [thumb_g2]
  Complex to Real-Imag10/1 -> [thumb_g1]

== system dx_hand_model/Thumb/Force Feedback ==
  Active : Subsystem
  Display10 : Display
  Gain : Gain  Gain=1/500
  g1 : Subsystem
  tag scope: ThumbForceReference=global
  wires:
  [CurrentThumbFlex] -> Gain/1
  Gain/1 -> g1/1(in)
  g1/1("out ") -> Display10/1, Active/1(in)
  Active/1(out) -> [ThumbForceReference]

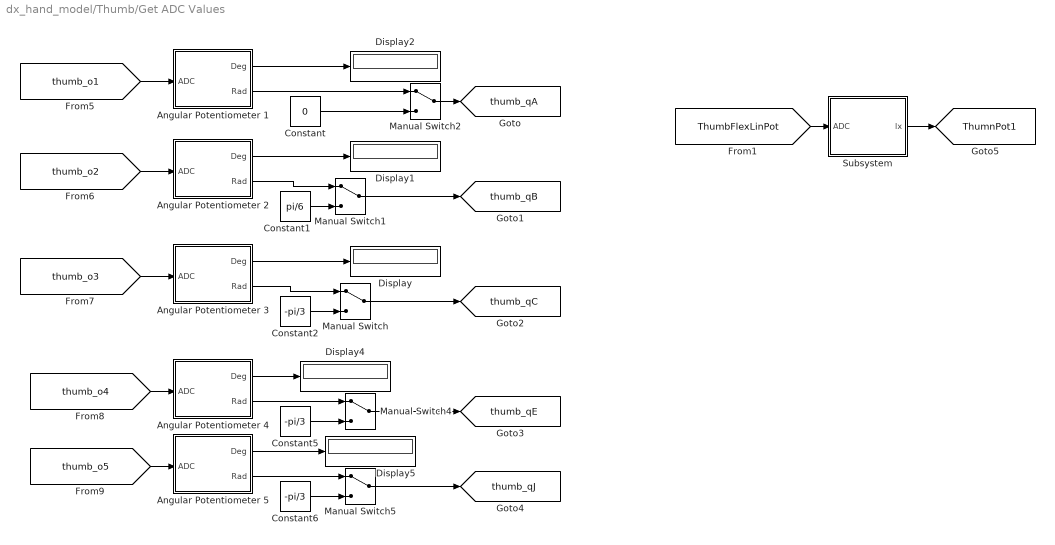
== system dx_hand_model/Thumb/Get ADC Values ==
  Angular Potentiometer 1 : Subsystem
  Angular Potentiometer 2 : Subsystem
  Angular Potentiometer 3 : Subsystem
  Angular Potentiometer 4 : Subsystem
  Angular Potentiometer 5 : Subsystem
  Constant : Constant  Value=0
  Constant1 : Constant  Value=pi/6
  Constant2 : Constant  Value=-pi/3
  Constant5 : Constant  Value=-pi/3
  Constant6 : Constant  Value=-pi/3
  Display{,1..2,4..5} (5 alike) : Display
  Manual Switch{,1..2,4..5} (5 alike) : ManualSwitch
  Subsystem : Subsystem
  tag scope: ThumnPot1=global, thumb_qA=global, thumb_qB=global, thumb_qC=global, thumb_qE=global, thumb_qJ=global
  wires:
  Constant5/1 -> Manual Switch4/2
  Manual Switch1/1 -> [thumb_qB]
  Angular Potentiometer 3/1(Deg) -> Display/1
  Manual Switch4/1 -> [thumb_qE]
  Constant6/1 -> Manual Switch5/2
  Angular Potentiometer 5/1(Deg) -> Display5/1
  Angular Potentiometer 3/2(Rad) -> Manual Switch/1
  Constant1/1 -> Manual Switch1/2
  [thumb_o1] -> Angular Potentiometer 1/1(ADC)
  [thumb_o4] -> Angular Potentiometer 4/1(ADC)
  [thumb_o3] -> Angular Potentiometer 3/1(ADC)
  Angular Potentiometer 1/2(Rad) -> Manual Switch2/1
  Constant/1 -> Manual Switch2/2
  Angular Potentiometer 2/2(Rad) -> Manual Switch1/1
  Angular Potentiometer 4/1(Deg) -> Display4/1
  Constant2/1 -> Manual Switch/2
  [thumb_o5] -> Angular Potentiometer 5/1(ADC)
  Angular Potentiometer 2/1(Deg) -> Display1/1
  Angular Potentiometer 1/1(Deg) -> Display2/1
  [thumb_o2] -> Angular Potentiometer 2/1(ADC)
  Manual Switch5/1 -> [thumb_qJ]
  Manual Switch2/1 -> [thumb_qA]
  Manual Switch/1 -> [thumb_qC]
  Angular Potentiometer 5/2(Rad) -> Manual Switch5/1
  Angular Potentiometer 4/2(Rad) -> Manual Switch4/1
  [ThumbFlexLinPot] -> Subsystem/1(ADC)
  Subsystem/1("lx ") -> [ThumnPot1]

== system dx_hand_model/Thumb/Get_from_ROS_param ==
  Get Parameter : robotlib/Get Parameter  SourceLibraryInfo=This block requires Robotics System Toolbox  ParameterSource=Specify your own  ParameterName=/hand_exo/thumb/CMCz  ParameterType=double  ParameterMaxArrayLength=16  ParameterInitialValue=-32.0  SampleTime=update_param  ShowErrorCodeOutput=on  ModelName=dx_hand_model  BlockId=ParamGet_dx_hand_model_3442
      settings: SourceProductName=Robotics System Toolbox  SourceProductBaseCode=RO
  Get Parameter1 : robotlib/Get Parameter  SourceLibraryInfo=This block requires Robotics System Toolbox  ParameterSource=Specify your own  ParameterName=/hand_exo/thumb/s1  ParameterType=double  ParameterMaxArrayLength=16  ParameterInitialValue=20.0  SampleTime=update_param  ShowErrorCodeOutput=on  ModelName=dx_hand_model  BlockId=ParamGet_dx_hand_model_3443
      settings: SourceProductName=Robotics System Toolbox  SourceProductBaseCode=RO
  Get Parameter2 : robotlib/Get Parameter  SourceLibraryInfo=This block requires Robotics System Toolbox  ParameterSource=Specify your own  ParameterName=/hand_exo/thumb/CMCy  ParameterType=double  ParameterMaxArrayLength=16  ParameterInitialValue=0.0  SampleTime=update_param  ShowErrorCodeOutput=on  ModelName=dx_hand_model  BlockId=ParamGet_dx_hand_model_3444
      settings: SourceProductName=Robotics System Toolbox  SourceProductBaseCode=RO
  Get Parameter3 : robotlib/Get Parameter  SourceLibraryInfo=This block requires Robotics System Toolbox  ParameterSource=Specify your own  ParameterName=/hand_exo/thumb/CMCx  ParameterType=double  ParameterMaxArrayLength=16  ParameterInitialValue=-10.0  SampleTime=update_param  ShowErrorCodeOutput=on  ModelName=dx_hand_model  BlockId=ParamGet_dx_hand_model_3445
      settings: SourceProductName=Robotics System Toolbox  SourceProductBaseCode=RO
  Get Parameter4 : robotlib/Get Parameter  SourceLibraryInfo=This block requires Robotics System Toolbox  ParameterSource=Specify your own  ParameterName=/hand_exo/thumb/l_meta  ParameterType=double  ParameterMaxArrayLength=16  ParameterInitialValue=50.0  SampleTime=update_param  ShowErrorCodeOutput=on  ModelName=dx_hand_model  BlockId=ParamGet_dx_hand_model_3446
      settings: SourceProductName=Robotics System Toolbox  SourceProductBaseCode=RO
  Get Parameter5 : robotlib/Get Parameter  SourceLibraryInfo=This block requires Robotics System Toolbox  ParameterSource=Specify your own  ParameterName=/hand_exo/thumb/s2  ParameterType=double  ParameterMaxArrayLength=16  ParameterInitialValue=20.0  SampleTime=update_param  ShowErrorCodeOutput=on  ModelName=dx_hand_model  BlockId=ParamGet_dx_hand_model_3454
      settings: SourceProductName=Robotics System Toolbox  SourceProductBaseCode=RO
  Get Parameter6 : robotlib/Get Parameter  SourceLibraryInfo=This block requires Robotics System Toolbox  ParameterSource=Specify your own  ParameterName=/hand_exo/thumb/l_dist  ParameterType=double  ParameterMaxArrayLength=16  ParameterInitialValue=30.0  SampleTime=update_param  ShowErrorCodeOutput=on  ModelName=dx_hand_model  BlockId=ParamGet_dx_hand_model_4055
      settings: SourceProductName=Robotics System Toolbox  SourceProductBaseCode=RO
  Mux : Mux  Inputs=3
  Subsystem : Subsystem
  Subsystem1 : Subsystem
  Subsystem2 : Subsystem
  Subsystem3 : Subsystem
  Subsystem4 : Subsystem
  Subsystem5 : Subsystem
  Subsystem6 : Subsystem
  Terminator{,1..6} (7 alike) : Terminator
  tag scope: thumb_CMC=global, thumb_l_dist=global, thumb_l_meta=global, thumb_s1=global, thumb_s2=global
  wires:
  Get Parameter/1 -> Subsystem2/1(In1)
  Get Parameter1/1 -> Subsystem3/1(In1)
  Get Parameter2/1 -> Subsystem1/1(In1)
  Get Parameter4/1 -> Subsystem4/1(In1)
  Get Parameter2/2 -> Terminator1/1
  Get Parameter4/2 -> Terminator4/1
  Get Parameter/2 -> Terminator2/1
  Get Parameter1/2 -> Terminator3/1
  Get Parameter3/2 -> Terminator/1
  Get Parameter5/2 -> Terminator5/1
  Get Parameter5/1 -> Subsystem5/1(In1)
  Mux/1 -> [thumb_CMC]
  Get Parameter3/1 -> Subsystem/1(In1)
  Subsystem/1(Out1) -> Mux/1
  Subsystem1/1(Out1) -> Mux/2
  Subsystem2/1(Out1) -> Mux/3
  Subsystem3/1(Out1) -> [thumb_s1]
  Subsystem4/1(Out1) -> [thumb_l_meta]
  Subsystem5/1(Out1) -> [thumb_s2]
  Subsystem6/1(Out1) -> [thumb_l_dist]
  Get Parameter6/2 -> Terminator6/1
  Get Parameter6/1 -> Subsystem6/1(In1)

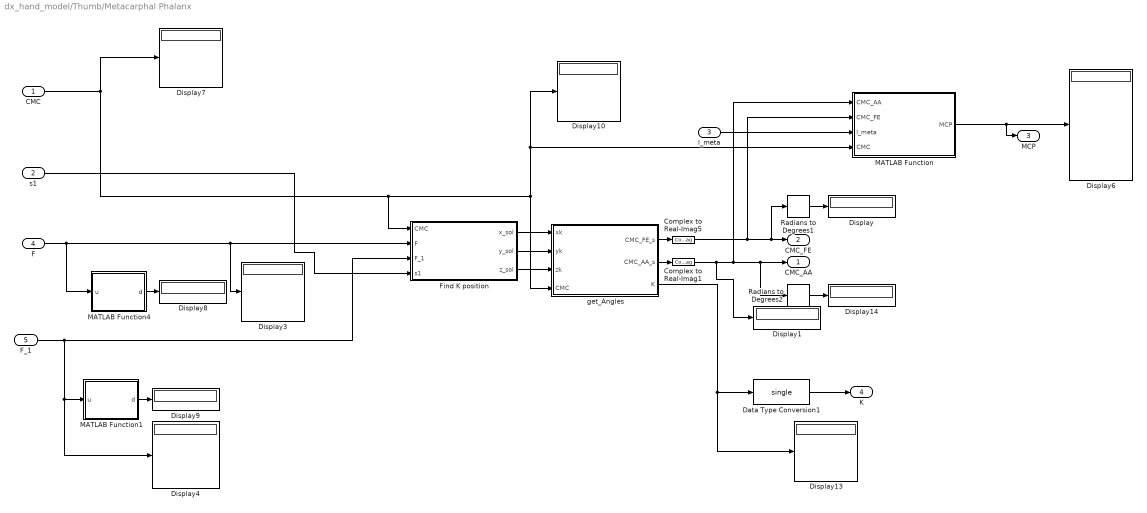
== system dx_hand_model/Thumb/Metacarphal Phalanx ==
  CMC : Inport
  s1 : Inport  Port=2
  l_meta : Inport  Port=3
  F : Inport  Port=4
  F_1 : Inport  Port=5
  Complex to Real-Imag1 : ComplexToRealImag  Output=Real
  Complex to Real-Imag5 : ComplexToRealImag  Output=Real
  Data Type Conversion1 : DataTypeConversion  OutDataTypeStr=single
  Display{,1,3..4,6..10,13..14} (11 alike) : Display
  Find K position : MATLAB Function  TreatAsAtomicUnit=on
  MATLAB Function : MATLAB Function  TreatAsAtomicUnit=on
  MATLAB Function1 : MATLAB Function  TreatAsAtomicUnit=on
  MATLAB Function4 : MATLAB Function  TreatAsAtomicUnit=on
  Radians to Degrees1 : simulink_extras/Transformations/Radians to Degrees
  Radians to Degrees2 : simulink_extras/Transformations/Radians to Degrees
  get_Angles : MATLAB Function  TreatAsAtomicUnit=on
  "CMC_AA " : Outport
  CMC_FE : Outport  Port=2
  MCP : Outport  Port=3
  K : Outport  Port=4
  wires:
  Find K position/2(y_sol) -> get_Angles/2(yk)
  Find K position/3(z_sol) -> get_Angles/3(zk)
  Find K position/1(x_sol) -> get_Angles/1(xk)
  CMC/1 -> Display7/1, Display10/1, MATLAB Function/4(CMC), get_Angles/4(CMC), Find K position/1(CMC)
  s1/1 -> Find K position/4(s1)
  l_meta/1 -> MATLAB Function/3(l_meta)
  get_Angles/2(CMC_AA_s) -> Complex to Real-Imag1/1
  get_Angles/1(CMC_FE_s) -> Complex to Real-Imag5/1
  MATLAB Function4/1(d) -> Display8/1
  F/1 -> MATLAB Function4/1(u), Find K position/2(F), Display3/1
  MATLAB Function1/1(d) -> Display9/1
  F_1/1 -> MATLAB Function1/1(u), Display4/1, Find K position/3(F_1)
  MATLAB Function/1(MCP) -> Display6/1, MCP/1
  get_Angles/3(K) -> Display13/1, Data Type Conversion1/1
  Radians to Degrees1/1 -> Display/1
  Radians to Degrees2/1 -> Display14/1
  Data Type Conversion1/1 -> K/1
  Complex to Real-Imag5/1 -> MATLAB Function/2(CMC_FE), Radians to Degrees1/1, CMC_FE/1
  Complex to Real-Imag1/1 -> Display1/1, MATLAB Function/1(CMC_AA), Radians to Degrees2/1, "CMC_AA "/1

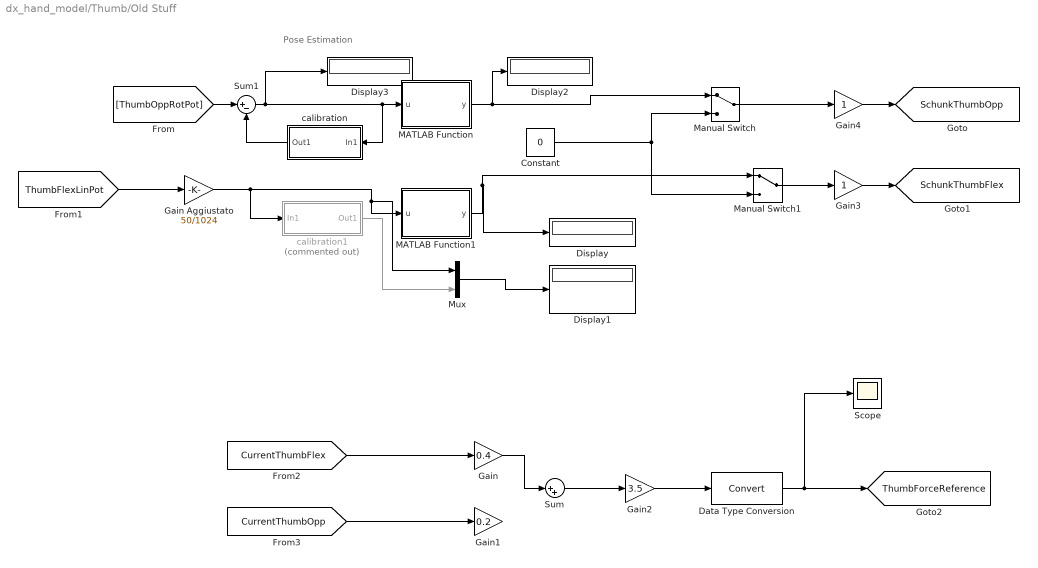
== system dx_hand_model/Thumb/Old Stuff ==
  note: Pose Estimation
  Constant : Constant  Value=0  OutDataTypeStr=single
  Data Type Conversion : DataTypeConversion
  Display{,1..3} (4 alike) : Display
  Gain : Gain  Gain=0.4
  Gain Aggiustato : Gain  Gain=50/1024
  Gain1 : Gain  Gain=0.2
  Gain2 : Gain  Gain=3.5
  Gain3 : Gain
  Gain4 : Gain
  MATLAB Function : MATLAB Function  TreatAsAtomicUnit=on
  MATLAB Function1 : MATLAB Function  TreatAsAtomicUnit=on
  Manual Switch : ManualSwitch
  Manual Switch1 : ManualSwitch
  Mux : Mux  Inputs=2
  Scope : Scope
  Sum : Sum  Inputs=|++
  Sum1 : Sum  Inputs=|+-
  calibration : Subsystem
  calibration1 : Subsystem  Commented=on
  tag scope: SchunkThumbFlex=global, SchunkThumbOpp=global, ThumbForceReference=global
  wires:
  MATLAB Function/1(y) -> Display2/1, Manual Switch/1
  Gain4/1 -> [SchunkThumbOpp]
  [ThumbFlexLinPot] -> Gain Aggiustato/1
  Sum/1 -> Gain2/1
  Data Type Conversion/1 -> Scope/1, [ThumbForceReference]
  Gain2/1 -> Data Type Conversion/1
  Gain3/1 -> [SchunkThumbFlex]
  Sum1/1 -> Display3/1, calibration/1(In1), MATLAB Function/1(u)
  Mux/1 -> Display1/1
  [CurrentThumbFlex] -> Gain/1
  MATLAB Function1/1(y) -> Manual Switch1/1, Display/1
  Manual Switch/1 -> Gain4/1
  Manual Switch1/1 -> Gain3/1
  [CurrentThumbOpp] -> Gain1/1
  Constant/1 -> Manual Switch1/2, Manual Switch/2
  calibration/1(Out1) -> Sum1/2
  Gain/1 -> Sum/1
  calibration1/1(Out1) -> Mux/2
  Gain Aggiustato/1 -> calibration1/1(In1), Mux/1, MATLAB Function1/1(u)
  [ThumbOppRotPot] -> Sum1/1

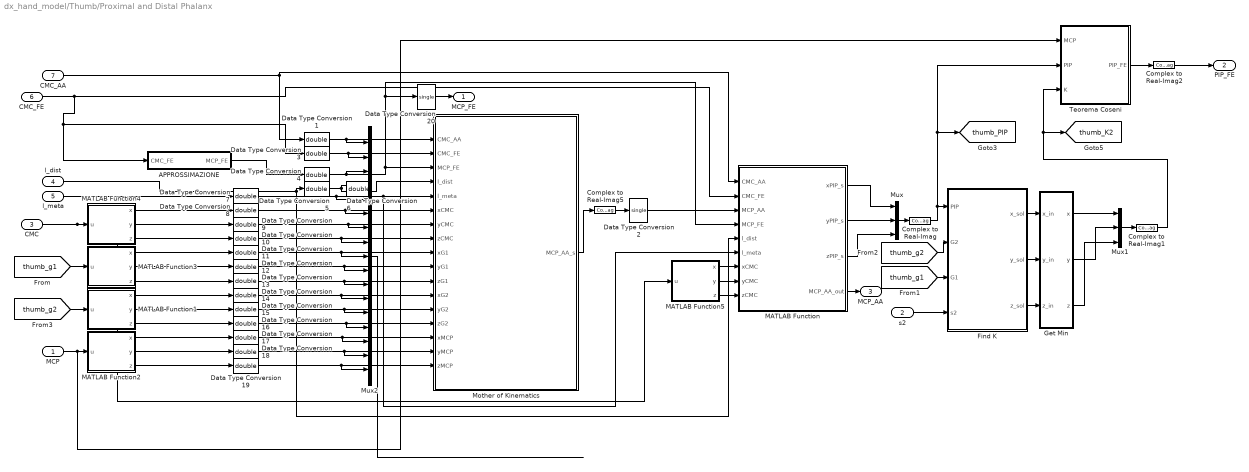
== system dx_hand_model/Thumb/Proximal and Distal Phalanx ==
  "MCP " : Inport
  s2 : Inport  Port=2
  CMC : Inport  Port=3
  l_dist : Inport  Port=4
  l_meta : Inport  Port=5
  CMC_FE : Inport  Port=6
  CMC_AA : Inport  Port=7
  APPROSSIMAZIONE : MATLAB Function  TreatAsAtomicUnit=on
  Complex to Real-Imag{,1..2,5} (4 alike) : ComplexToRealImag  Output=Real
  Data Type Conversion{1,3..19} (18 alike) : DataTypeConversion  OutDataTypeStr=double
  Data Type Conversion2 : DataTypeConversion  OutDataTypeStr=single
  Data Type Conversion20 : DataTypeConversion  OutDataTypeStr=single
  Find K : MATLAB Function  TreatAsAtomicUnit=on
  Get Min : MATLAB Function  TreatAsAtomicUnit=on
  MATLAB Function : MATLAB Function  TreatAsAtomicUnit=on
  MATLAB Function1 : MATLAB Function  TreatAsAtomicUnit=on
  MATLAB Function2 : MATLAB Function  TreatAsAtomicUnit=on
  MATLAB Function3 : MATLAB Function  TreatAsAtomicUnit=on
  MATLAB Function4 : MATLAB Function  TreatAsAtomicUnit=on
  MATLAB Function5 : MATLAB Function  TreatAsAtomicUnit=on
  Mother of Kinematics : MATLAB Function  TreatAsAtomicUnit=on
  Mux : Mux  Inputs=3
  Mux1 : Mux  Inputs=3
  Mux2 : Mux  Inputs=17
  Teorema Coseni : MATLAB Function  TreatAsAtomicUnit=on
  MCP_FE : Outport
  PIP_FE : Outport  Port=2
  MCP_AA : Outport  Port=3
  tag scope: thumb_K2=global, thumb_PIP=global
  wires:
  MATLAB Function2/3(z) -> Data Type Conversion19/1
  MATLAB Function2/2(y) -> Data Type Conversion18/1
  MATLAB Function2/1(x) -> Data Type Conversion17/1
  MATLAB Function1/2(y) -> Data Type Conversion15/1
  MATLAB Function1/3(z) -> Data Type Conversion16/1
  MATLAB Function3/3(z) -> Data Type Conversion13/1
  MATLAB Function3/2(y) -> Data Type Conversion12/1
  MATLAB Function3/1(x) -> Data Type Conversion11/1
  MATLAB Function4/3(z) -> Data Type Conversion10/1
  MATLAB Function4/2(y) -> Data Type Conversion9/1
  MATLAB Function4/1(x) -> Data Type Conversion8/1
  l_meta/1 -> Data Type Conversion7/1
  l_dist/1 -> MATLAB Function/5(l_dist), Data Type Conversion5/1
  CMC_FE/1 -> MATLAB Function/2(CMC_FE), Data Type Conversion3/1, APPROSSIMAZIONE/1(CMC_FE)
  CMC_AA/1 -> Data Type Conversion1/1, MATLAB Function/1(CMC_AA)
  APPROSSIMAZIONE/1(MCP_FE) -> Data Type Conversion4/1
  MATLAB Function5/3(z) -> MATLAB Function/9(zCMC)
  MATLAB Function5/2(y) -> MATLAB Function/8(yCMC)
  MATLAB Function5/1(x) -> MATLAB Function/7(xCMC)
  CMC/1 -> MATLAB Function5/1(u), MATLAB Function4/1(u)
  s2/1 -> Find K/4(s2)
  Mux/1 -> Complex to Real-Imag/1
  Complex to Real-Imag/1 -> [thumb_PIP], Teorema Coseni/2(PIP), Find K/1(PIP)
  MATLAB Function/1(xPIP_s) -> Mux/1
  MATLAB Function/2(yPIP_s) -> Mux/2
  MATLAB Function/3(zPIP_s) -> Mux/3
  Teorema Coseni/1(PIP_FE) -> Complex to Real-Imag2/1
  Get Min/3(z) -> Mux1/3
  Get Min/2(y) -> Mux1/2
  Mux1/1 -> Complex to Real-Imag1/1
  Get Min/1(x) -> Mux1/1
  Complex to Real-Imag1/1 -> [thumb_K2], Teorema Coseni/3(K)
  Find K/2(y_sol) -> Get Min/2(y_in)
  Find K/1(x_sol) -> Get Min/1(x_in)
  Find K/3(z_sol) -> Get Min/3(z_in)
  [thumb_g1] -> MATLAB Function3/1(u)
  [thumb_g1] -> Find K/3(G1)
  [thumb_g2] -> MATLAB Function1/1(u)
  [thumb_g2] -> Find K/2(G2)
  MATLAB Function1/1(x) -> Data Type Conversion14/1
  Mux2/1 -> ?
  Data Type Conversion1/1 -> Mux2/1, Mother of Kinematics/1(CMC_AA)
  Data Type Conversion3/1 -> Mux2/2, Mother of Kinematics/2(CMC_FE)
  Data Type Conversion4/1 -> Mux2/3, Mother of Kinematics/3(MCP_FE), MATLAB Function/4(MCP_FE), Data Type Conversion20/1
  Data Type Conversion5/1 -> Mother of Kinematics/4(l_dist), Mux2/4
  Data Type Conversion7/1 -> Mux2/5, Mother of Kinematics/5(l_meta), MATLAB Function/6(l_meta)
  Data Type Conversion8/1 -> Mux2/6, Mother of Kinematics/6(xCMC)
  Data Type Conversion9/1 -> Mux2/7, Mother of Kinematics/7(yCMC)
  Data Type Conversion10/1 -> Mux2/8, Mother of Kinematics/8(zCMC)
  Data Type Conversion11/1 -> Mux2/9, Mother of Kinematics/9(xG1)
  Data Type Conversion12/1 -> Mux2/10, Mother of Kinematics/10(yG1)
  Data Type Conversion13/1 -> Mux2/11, Mother of Kinematics/11(zG1)
  Data Type Conversion14/1 -> Mux2/12, Mother of Kinematics/12(xG2)
  Data Type Conversion15/1 -> Mux2/13, Mother of Kinematics/13(yG2)
  Data Type Conversion16/1 -> Mux2/14, Mother of Kinematics/14(zG2)
  Data Type Conversion17/1 -> Mux2/15, Mother of Kinematics/15(xMCP)
  "MCP "/1 -> Teorema Coseni/1(MCP), MATLAB Function2/1(u)
  Data Type Conversion18/1 -> Mux2/16, Mother of Kinematics/16(yMCP)
  Data Type Conversion19/1 -> Mux2/17, Mother of Kinematics/17(zMCP)
  Complex to Real-Imag5/1 -> Data Type Conversion2/1
  Mother of Kinematics/1(MCP_AA_s) -> Complex to Real-Imag5/1
  Data Type Conversion20/1 -> MCP_FE/1
  Complex to Real-Imag2/1 -> PIP_FE/1
  MATLAB Function/4(MCP_AA_out) -> MCP_AA/1
  Data Type Conversion2/1 -> MATLAB Function/3(MCP_AA)

== system dx_hand_model/Thumb/Study Gravity Compensation ==
  Constant3 : Constant
  Constant4 : Constant  Value=0
  Data Type Conversion1 : DataTypeConversion  OutDataTypeStr=single
  Manual Switch3 : ManualSwitch
  Subsystem2 : Subsystem
  wires:
  Constant4/1 -> Manual Switch3/1
  [ThumbForce] -> Subsystem2/2(In2)
  Constant3/1 -> Manual Switch3/2
  Manual Switch3/1 -> Subsystem2/Enable
  Data Type Conversion1/1 -> Subsystem2/1(In1)
  [thumb_qA] -> Data Type Conversion1/1

== system dx_hand_model/Thumb/ToSchunk ==
  Data Type Conversion2 : DataTypeConversion  OutDataTypeStr=double
  Degrees to Radians2 : simulink_extras/Transformations/Degrees to Radians
  Display{,1..3} (4 alike) : Display
  Gain : Gain  Gain=1/1.44889
  Radians to Degrees3 : simulink_extras/Transformations/Radians to Degrees
  Radians to Degrees5 : simulink_extras/Transformations/Radians to Degrees
  Set Parameter : robotlib/Set Parameter  SourceLibraryInfo=This block requires Robotics System Toolbox  ParameterSource=Specify your own  ParameterName=/hand_exo/thumb/offset/get_opp  ParameterType=double  ModelName=dx_hand_model  BlockId=ParamSet_dx_hand_model_4969
      settings: SourceProductName=Robotics System Toolbox  SourceProductBaseCode=RO
  Subsystem : Subsystem
  Subsystem1 : Subsystem
  Sum : Sum  Inputs=|++
  Sum1 : Sum  Inputs=|++
  Sum4 : Sum  Inputs=|+-
  Sum5 : Sum  Inputs=|++
  THUMB_FLEX : Outport
  THUMB_OPP : Outport  Port=2
  tag scope: SchunkThumbFlex=global, SchunkThumbOpp=global
  wires:
  Radians to Degrees3/1 -> THUMB_FLEX/1, Display/1
  [thumb_CMC_AA] -> Sum5/1
  Radians to Degrees5/1 -> THUMB_OPP/1, Display3/1
  [thumb_PIP_FE] -> Gain/1
  [thumb_MCP_AA] -> Sum5/2
  Gain/1 -> Sum4/1
  Degrees to Radians2/1 -> Sum4/2
  Subsystem1/1(offset) -> Degrees to Radians2/1
  [thumb_CMC_FE] -> Sum1/1
  [thumb_PIP_FE] -> Sum1/2
  Sum1/1 -> Display1/1, Radians to Degrees3/1, [SchunkThumbFlex]
  Sum/1 -> Radians to Degrees5/1, Display2/1, [SchunkThumbOpp]
  Sum5/1 -> Data Type Conversion2/1, Sum/1
  Subsystem/1(offset) -> Sum/2
  Data Type Conversion2/1 -> Set Parameter/1

== system dx_hand_model/Get From Schunk/Get positions/Get Efforts ==
  <Effort> : Inport
  Data Type Conversion{1..4} (4 alike) : DataTypeConversion  OutDataTypeStr=single
  Demux1 : Demux  Outputs=10
  Display2 : Display
  Selector1 : Selector  IndexOptions=Index vector (dialog)  Indices=[2 3 4 5 6 7 8 9 10 11]  OutputSizes=1
  tag scope: effort_IndexDistal=global, effort_IndexProxi=global, effort_MiddleDistal=global, effort_MiddleProxi=global
  wires:
  Data Type Conversion4/1 -> [effort_MiddleProxi]
  Data Type Conversion3/1 -> [effort_MiddleDistal]
  <Effort>/1 -> Selector1/1
  Selector1/1 -> Display2/1, Demux1/1
  Demux1/5 -> Data Type Conversion4/1
  Demux1/4 -> Data Type Conversion3/1
  Data Type Conversion2/1 -> [effort_IndexProxi]
  Data Type Conversion1/1 -> [effort_IndexDistal]
  Demux1/3 -> Data Type Conversion2/1
  Demux1/2 -> Data Type Conversion1/1
